simulink model "Mostar_RaPId"  (Simulink 10.1)
settings: Solver=ode45  StartTime=0  StopTime=4.5  FixedStep=0.01  RelTol=0.001  EnableMultiTasking=on
libraries: fmu_me_lib x1
settings Model: Creator=Tin Rabuzin  LastModifiedBy=meagh
settings DataIOCC: LimitDataPoints=on  OutputSaveName=simout  OutputOption=SpecifiedOutputTimes  OutputTimes=[0:0.005:4.5]
settings OptimizationCC: ExpressionDepthLimit=2147483647
settings DebuggingCC: StateNameClashWarn=warning
settings GRTTargetCC: CombineOutputUpdateFcns=on  GRTInterface=off

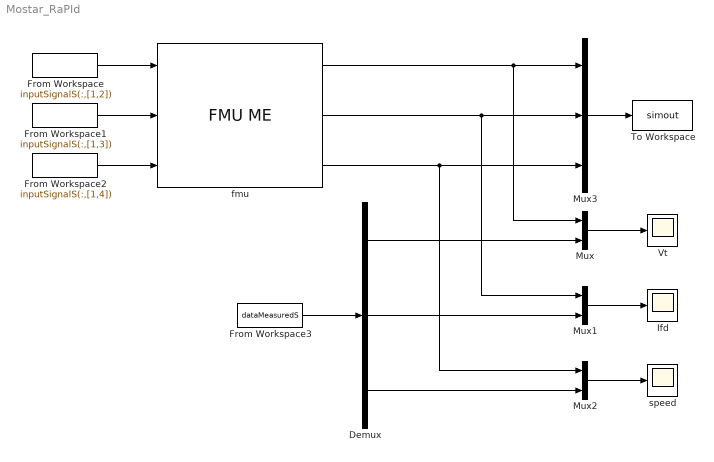
== system Mostar_RaPId ==
  Demux : Demux  Outputs=3
  From Workspace : FromWorkspace  VariableName=inputSignalS(:,[1,2])
  From Workspace1 : FromWorkspace  VariableName=inputSignalS(:,[1,3])
  From Workspace2 : FromWorkspace  VariableName=inputSignalS(:,[1,4])
  From Workspace3 : FromWorkspace  VariableName=dataMeasuredS
  Ifd : Scope
  Mux : Mux  Inputs=2
  Mux1 : Mux  Inputs=2
  Mux2 : Mux  Inputs=2
  Mux3 : Mux  Inputs=3
  To Workspace : ToWorkspace  VariableName=simout  SaveFormat=Structure With Time  SampleTime=-1
  Vt : Scope
  fmu : fmu_me_lib/FMU ME  Description=Simulates an FMU for Model Exchange 1.0 or Model Exchange 2.0.  dummy=0
  speed : Scope
  wires:
  fmu/2 -> Mux1/1, Mux3/2
  fmu/1 -> Mux/1, Mux3/1
  fmu/3 -> Mux2/1, Mux3/3
  From Workspace1/1 -> fmu/2
  From Workspace2/1 -> fmu/3
  From Workspace/1 -> fmu/1
  Mux3/1 -> To Workspace/1
  Demux/3 -> Mux2/2
  From Workspace3/1 -> Demux/1
  Mux/1 -> Vt/1
  Demux/1 -> Mux/2
  Mux1/1 -> Ifd/1
  Demux/2 -> Mux1/2
  Mux2/1 -> speed/1
